simulink model "fuzzy2_3064"  (R2016b)
settings: Solver=VariableStepAuto  StartTime=0.0  StopTime=10.0  RelTol=1e-3
libraries: fuzblock x1
settings Model: Creator=student  LastModifiedBy=student

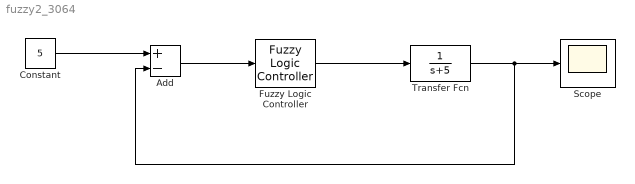
== system fuzzy2_3064 ==
  Add : Sum  Inputs=+-
  Constant : Constant  Value=5
  Fuzzy Logic Controller : fuzblock/Fuzzy Logic  Controller  fis='lab4_2.fis'
  Scope : Scope
  Transfer Fcn : TransferFcn  Denominator=[1 5]
  wires:
  Fuzzy Logic Controller/1 -> Transfer Fcn/1
  Add/1 -> Fuzzy Logic Controller/1
  Constant/1 -> Add/1
  Transfer Fcn/1 -> Add/2, Scope/1
